simulink model "Siemens_Shock_discrete_exp"  (R2019b)
settings: Solver=FixedStepDiscrete  StartTime=0.0  StopTime=inf  FixedStep=sample_time_calc  RelTol=1e-3  EnableMultiTasking=on
undefined symbols (not defined in the file): DiscIntNeverNeededParam, dK, g, h_Auflage, J_Kugel, magnitude, max_angle, sample_time_calc
libraries: simulink x1
settings Model: Creator=berroth  LastModifiedBy=Siemens
settings DataIOCC: LimitDataPoints=on  SaveFormat=Array  SaveOutput=off  SaveTime=off  ReturnWorkspaceOutputs=off
settings OptimizationCC: ExpressionDepthLimit=2147483647
settings DebuggingCC: UnderspecifiedInitializationDetection=Classic  MergeDetectMultiDrivingBlocksExec=none  SolverPrmCheckMsg=warning  FcnCallInpInsideContextMsg=warning  StateNameClashWarn=warning  SFUnexpectedBacktrackingDiag=warning  SFNoUnconditionalDefaultTransitionDiag=warning  SFExecutionAtInitializationDiag=none  ArithmeticOperatorsInVariantConditions=warning
settings HardwareCC: ProdBitPerPointer=32  ProdBitPerSizeT=32  ProdBitPerPtrDiffT=32  ProdLargestAtomicFloat=None  ProdWordSize=32  ProdLongLongMode=on  ProdHWDeviceType=Intel->x86/Pentium
settings ModelReferenceCC: PropagateSignalLabelsOutOfModel=off
settings SFSimCC: SimUseLocalCustomCode=off  MATLABDynamicMemAlloc=off  CustomCodeUndefinedFunction=UseInterfaceOnly
settings RTWCC: Description=Generic Real-Time Target  GenCodeOnly=on  PackageGeneratedCodeAndArtifacts=on  PackageName=shock_sensor  RTWUseLocalCustomCode=off  Toolchain=Microsoft Visual C++ 2015 v14.0 | nmake (64-bit Windows)  TargetLang=C++
settings CodeAppCC: StateflowObjectComments=on
settings GRTTargetCC: TargetLangStandard=C89/C90 (ANSI)  MatFileLogging=off  MultiInstanceERTCode=on  CodeInterfacePackaging=C++ class  RTWCAPISignals=on  RTWCAPIParams=on  RTWCAPIStates=on  RTWCAPIRootIO=on
settings ConfigComp: CovMetricSettings=dw  CovHtmlReporting=on  CovSaveCumulativeToWorkspaceVar=on  CovSaveSingleToWorkspaceVar=on  CovExternalEMLEnable=off  CovSFcnEnable=off

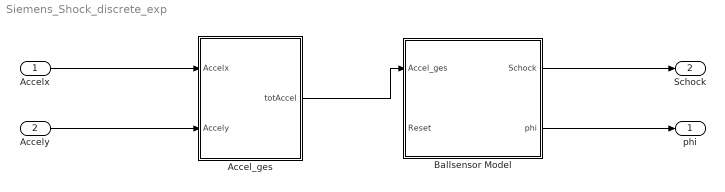
== system Siemens_Shock_discrete_exp ==
  Accelx : Inport
  Accely : Inport  Port=2
  Accel_ges : Subsystem
  Ballsensor Model : Subsystem
  phi : Outport  VectorParamsAs1DForOutWhenUnconnected=off
  Schock : Outport  Port=2  VectorParamsAs1DForOutWhenUnconnected=off
  wires:
  Accel_ges/1(totAccel) -> Ballsensor Model/1(Accel_ges)
  Ballsensor Model/1(Schock) -> Schock/1
  Ballsensor Model/2(phi) -> phi/1
  Accelx/1 -> Accel_ges/1(Accelx)
  Accely/1 -> Accel_ges/2(Accely)

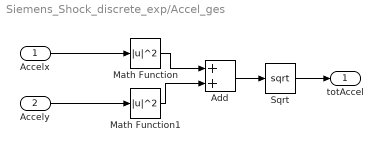
== system Siemens_Shock_discrete_exp/Accel_ges ==
  Accelx : Inport
  Accely : Inport  Port=2
  Add : Sum  SampleTime=sample_time_calc
  Math Function : Math  Operator=magnitude^2  SampleTime=sample_time_calc  SaturateOnIntegerOverflow=on
  Math Function1 : Math  Operator=magnitude^2  SampleTime=sample_time_calc  SaturateOnIntegerOverflow=on
  Sqrt : Sqrt  SampleTime=sample_time_calc  SaturateOnIntegerOverflow=on
  totAccel : Outport  VectorParamsAs1DForOutWhenUnconnected=off
  wires:
  Accelx/1 -> Math Function/1
  Accely/1 -> Math Function1/1
  Sqrt/1 -> totAccel/1
  Math Function/1 -> Add/1
  Math Function1/1 -> Add/2
  Add/1 -> Sqrt/1

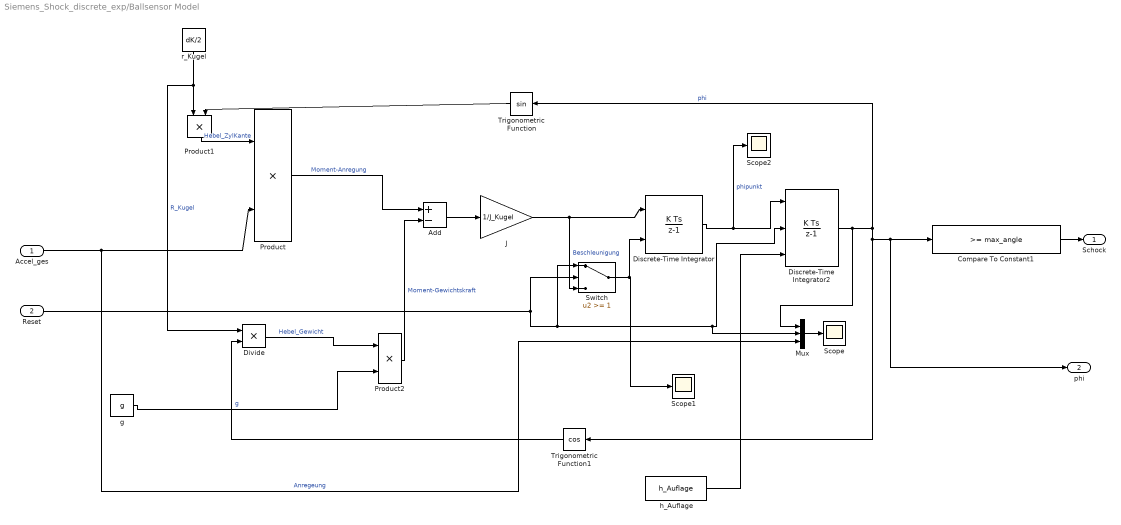
== system Siemens_Shock_discrete_exp/Ballsensor Model ==
  Accel_ges : Inport
  Reset : Inport  Port=2
  Add : Sum  Inputs=+-  SampleTime=sample_time_calc
  Compare To Constant1 : simulink/Logic and Bit Operations/Compare To Constant  relop=>=  const=max_angle  OutDataTypeStr=uint8
  Discrete-Time Integrator : DiscreteIntegrator  ExternalReset=rising  SampleTime=sample_time_calc  ICPrevOutput=DiscIntNeverNeededParam  ICPrevScaledInput=DiscIntNeverNeededParam
  Discrete-Time Integrator2 : DiscreteIntegrator  ExternalReset=level  InitialConditionSource=external  SampleTime=sample_time_calc  LimitOutput=on  UpperSaturationLimit=pi  LowerSaturationLimit=h_Auflage  ICPrevOutput=DiscIntNeverNeededParam  ICPrevScaledInput=DiscIntNeverNeededParam
  Divide : Product  Inputs=**  SampleTime=sample_time_calc
  J : Gain  Gain=1/J_Kugel  SampleTime=sample_time_calc
  Mux : Mux  Inputs=3
  Product : Product  SampleTime=sample_time_calc  RndMeth=Zero
  Product1 : Product  SampleTime=sample_time_calc  RndMeth=Zero
  Product2 : Product  SampleTime=sample_time_calc  RndMeth=Zero
  Scope : Scope
  Scope1 : Scope
  Scope2 : Scope
  Switch : Switch  Threshold=1
  Trigonometric Function : Trigonometry  SampleTime=sample_time_calc
  Trigonometric Function1 : Trigonometry  Operator=cos  SampleTime=sample_time_calc
  g : Constant  Value=g
  h_Auflage : Constant  Value=h_Auflage  SampleTime=sample_time_calc
  r_Kugel : Constant  Value=dK/2
  Schock : Outport  VectorParamsAs1DForOutWhenUnconnected=off
  phi : Outport  Port=2  VectorParamsAs1DForOutWhenUnconnected=off
  wires:
  Trigonometric Function1/1 -> Divide/2
  Mux/1 -> Scope/1
  Reset/1 -> Switch/1, Discrete-Time Integrator2/2, Mux/2, Switch/2
  Switch/1 -> Discrete-Time Integrator/2, Scope1/1
  Trigonometric Function/1 -> Product1/2
  Discrete-Time Integrator/1 -> Scope2/1, Discrete-Time Integrator2/1  "phipunkt"
  Compare To Constant1/1 -> Schock/1
  h_Auflage/1 -> Discrete-Time Integrator2/3
  Divide/1 -> Product2/1  "Hebel_Gewicht"
  Product/1 -> Add/1  "Moment-Anregung"
  Add/1 -> J/1
  Accel_ges/1 -> Mux/3, Product/2  "Anregeung"
  r_Kugel/1 -> Product1/1, Divide/1  "R_Kugel"
  Discrete-Time Integrator2/1 -> Mux/1, Compare To Constant1/1, phi/1, Trigonometric Function1/1, Trigonometric Function/1  "phi"
  Product1/1 -> Product/1  "Hebel_ZylKante"
  Product2/1 -> Add/2  "Moment-Gewichtskraft"
  g/1 -> Product2/2  "g"
  J/1 -> Switch/3, Discrete-Time Integrator/1  "Beschleunigung"
